simulink model "notch_filter"  (R2023a)
settings: configuration reference "config" (kept outside this file)
model workspace (MAT data in the model file):
  damp = Simulink.Parameter
  damp.Value = 10
  damp.DataType = 'double'
  damp.Complexity = 'real'
  damp.Dimensions = [1 1]
  dt = Simulink.Parameter
  dt.Value = 0.0001
  dt.DataType = 'double'
  dt.Complexity = 'real'
  dt.Dimensions = [1 1]
  freq = Simulink.Parameter
  freq.Value = 439
  freq.DataType = 'double'
  freq.Complexity = 'real'
  freq.Dimensions = [1 1]
  gmin = Simulink.Parameter
  gmin.Value = 100
  gmin.DataType = 'double'
  gmin.Complexity = 'real'
  gmin.Dimensions = [1 1]
settings Model: DataDictionary=model_config.sldd  ParameterArgumentNames=damp,dt,freq,gmin  Creator=GQR  LastModifiedBy=Administrator
settings ConfigSetRef: SourceName=config

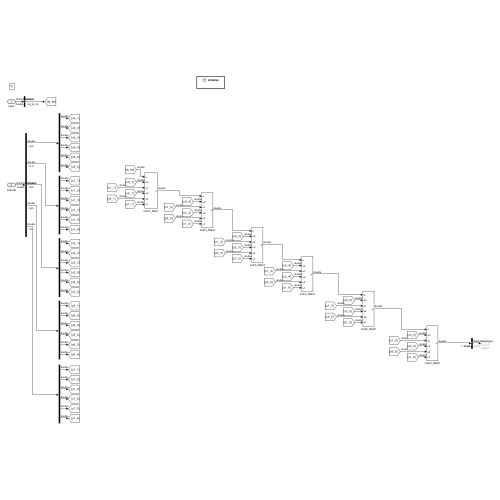
[thumbnail: Simulink's stored preview of the top-level diagram]
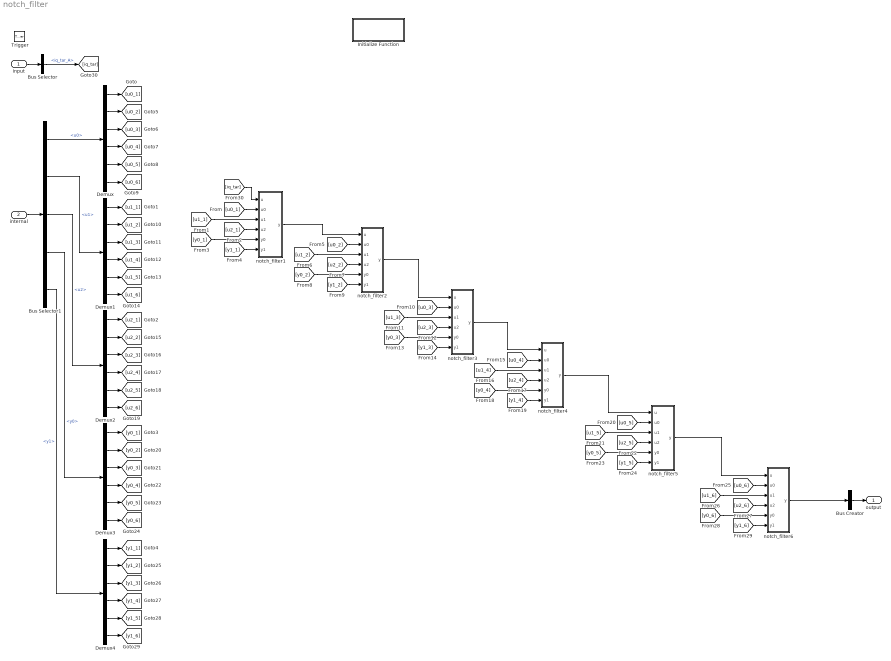
== system notch_filter ==
  input : Inport  OutDataTypeStr=Bus: NotchFilterInput  BusOutputAsStruct=on
  internal : Inport  Port=2  OutDataTypeStr=Bus: NotchFilterInternal  BusOutputAsStruct=on
  Trigger : TriggerPort  TriggerType=function-call  VariantControl=(inherit)  PortDimensions=1
  Bus Creator : BusCreator  Inputs=1  OutDataTypeStr=Bus: NotchFilterOutput  NonVirtualBus=on
      settings: InheritFromInputs=off
  Bus Selector : BusSelector  OutputSignals=iq_tar_A
  Bus Selector1 : BusSelector  OutputSignals=u0,u1,u2,y0,y1
  Demux{,1..4} (5 alike) : Demux  Outputs=6
  Initialize Function : Subsystem  TreatAsAtomicUnit=on
  notch_filter1 : Subsystem
  notch_filter2 : Subsystem
  notch_filter3 : Subsystem
  notch_filter4 : Subsystem
  notch_filter5 : Subsystem
  notch_filter6 : Subsystem
  output : Outport  OutDataTypeStr=Bus: NotchFilterOutput  BusOutputAsStruct=on
      settings: EnsureOutportIsVirtual=on
  wires:
  Demux4/6 -> [y1_6]
  Demux4/5 -> [y1_5]
  Demux1/1 -> [u1_1]
  internal/1 -> Bus Selector1/1
  Bus Selector1/5 -> Demux4/1  "<y1>"
  Demux2/2 -> [u2_2]
  input/1 -> Bus Selector/1
  Bus Selector1/4 -> Demux3/1  "<y0>"
  Bus Selector1/1 -> Demux/1  "<u0>"
  Bus Selector1/2 -> Demux1/1  "<u1>"
  Demux1/3 -> [u1_3]
  Bus Selector1/3 -> Demux2/1  "<u2>"
  Demux1/2 -> [u1_2]
  [u0_1] -> notch_filter1/2(u0)
  [u1_1] -> notch_filter1/3(u1)
  Bus Creator/1 -> output/1
  [u2_1] -> notch_filter1/4(u2)
  Demux3/6 -> [y0_6]
  Demux/2 -> [u0_2]
  [y1_1] -> notch_filter1/6(y1)
  [y0_1] -> notch_filter1/5(y0)
  Demux/1 -> [u0_1]
  Demux/3 -> [u0_3]
  Demux/4 -> [u0_4]
  Demux/5 -> [u0_5]
  Demux/6 -> [u0_6]
  Demux1/4 -> [u1_4]
  Demux1/5 -> [u1_5]
  Demux1/6 -> [u1_6]
  Demux2/6 -> [u2_6]
  Demux2/5 -> [u2_5]
  Demux2/1 -> [u2_1]
  Demux2/4 -> [u2_4]
  Demux2/3 -> [u2_3]
  Demux3/1 -> [y0_1]
  Demux3/3 -> [y0_3]
  Demux3/2 -> [y0_2]
  Demux3/5 -> [y0_5]
  Demux3/4 -> [y0_4]
  Demux4/2 -> [y1_2]
  Demux4/1 -> [y1_1]
  Demux4/4 -> [y1_4]
  Demux4/3 -> [y1_3]
  [y0_2] -> notch_filter2/5(y0)
  [y1_2] -> notch_filter2/6(y1)
  [u2_2] -> notch_filter2/4(u2)
  [u1_2] -> notch_filter2/3(u1)
  [u0_2] -> notch_filter2/2(u0)
  notch_filter1/1(y) -> notch_filter2/1(u)
  [u0_3] -> notch_filter3/2(u0)
  [u1_3] -> notch_filter3/3(u1)
  [u2_3] -> notch_filter3/4(u2)
  [y1_3] -> notch_filter3/6(y1)
  [y0_3] -> notch_filter3/5(y0)
  notch_filter2/1(y) -> notch_filter3/1(u)
  [y0_4] -> notch_filter4/5(y0)
  [y1_4] -> notch_filter4/6(y1)
  [u2_4] -> notch_filter4/4(u2)
  [u1_4] -> notch_filter4/3(u1)
  [u0_4] -> notch_filter4/2(u0)
  notch_filter3/1(y) -> notch_filter4/1(u)
  [u0_5] -> notch_filter5/2(u0)
  [u1_5] -> notch_filter5/3(u1)
  [u2_5] -> notch_filter5/4(u2)
  [y1_5] -> notch_filter5/6(y1)
  [y0_5] -> notch_filter5/5(y0)
  notch_filter4/1(y) -> notch_filter5/1(u)
  notch_filter5/1(y) -> notch_filter6/1(u)
  [y0_6] -> notch_filter6/5(y0)
  [y1_6] -> notch_filter6/6(y1)
  [u2_6] -> notch_filter6/4(u2)
  [u1_6] -> notch_filter6/3(u1)
  [u0_6] -> notch_filter6/2(u0)
  notch_filter6/1(y) -> Bus Creator/1
  Bus Selector/1 -> [iq_tar]  "<iq_tar_A>"
  [iq_tar] -> notch_filter1/1(u)

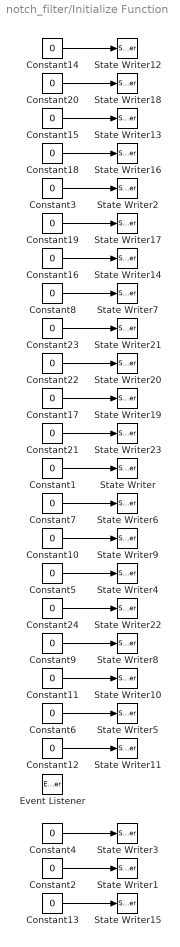
== system notch_filter/Initialize Function ==
  Constant{1..24} (24 alike) : Constant  Value=0  OutDataTypeStr=single
  Event Listener : EventListener  DisableCoverage=on  EventName=reset
  State Writer : StateWriter  StateOwnerBlock=../../notch_filter1/Delay  StateName=u_last
  State Writer1 : StateWriter  StateOwnerBlock=../../notch_filter1/Delay1  StateName=u_last
  State Writer10 : StateWriter  StateOwnerBlock=../../notch_filter3/Delay1  StateName=u_last
  State Writer11 : StateWriter  StateOwnerBlock=../../notch_filter3/Delay2  StateName=y_last
  State Writer12 : StateWriter  StateOwnerBlock=../../notch_filter4/Delay1  StateName=u_last
  State Writer13 : StateWriter  StateOwnerBlock=../../notch_filter4/Delay2  StateName=y_last
  State Writer14 : StateWriter  StateOwnerBlock=../../notch_filter4/Delay  StateName=u_last
  State Writer15 : StateWriter  StateOwnerBlock=../../notch_filter4/Delay3  StateName=y_last
  State Writer16 : StateWriter  StateOwnerBlock=../../notch_filter5/Delay1  StateName=u_last
  State Writer17 : StateWriter  StateOwnerBlock=../../notch_filter5/Delay2  StateName=y_last
  State Writer18 : StateWriter  StateOwnerBlock=../../notch_filter5/Delay  StateName=u_last
  State Writer19 : StateWriter  StateOwnerBlock=../../notch_filter5/Delay3  StateName=y_last
  State Writer2 : StateWriter  StateOwnerBlock=../../notch_filter1/Delay2  StateName=y_last
  State Writer20 : StateWriter  StateOwnerBlock=../../notch_filter6/Delay1  StateName=u_last
  State Writer21 : StateWriter  StateOwnerBlock=../../notch_filter6/Delay2  StateName=y_last
  State Writer22 : StateWriter  StateOwnerBlock=../../notch_filter6/Delay  StateName=u_last
  State Writer23 : StateWriter  StateOwnerBlock=../../notch_filter6/Delay3  StateName=y_last
  State Writer3 : StateWriter  StateOwnerBlock=../../notch_filter1/Delay3  StateName=y_last
  State Writer4 : StateWriter  StateOwnerBlock=../../notch_filter2/Delay  StateName=u_last
  State Writer5 : StateWriter  StateOwnerBlock=../../notch_filter2/Delay3  StateName=y_last
  State Writer6 : StateWriter  StateOwnerBlock=../../notch_filter2/Delay1  StateName=u_last
  State Writer7 : StateWriter  StateOwnerBlock=../../notch_filter2/Delay2  StateName=y_last
  State Writer8 : StateWriter  StateOwnerBlock=../../notch_filter3/Delay  StateName=u_last
  State Writer9 : StateWriter  StateOwnerBlock=../../notch_filter3/Delay3  StateName=y_last
  wires:
  Constant15/1 -> State Writer13/1
  Constant12/1 -> State Writer11/1
  Constant14/1 -> State Writer12/1
  Constant20/1 -> State Writer18/1
  Constant18/1 -> State Writer16/1
  Constant3/1 -> State Writer2/1
  Constant8/1 -> State Writer7/1
  Constant19/1 -> State Writer17/1
  Constant16/1 -> State Writer14/1
  Constant23/1 -> State Writer21/1
  Constant22/1 -> State Writer20/1
  Constant17/1 -> State Writer19/1
  Constant21/1 -> State Writer23/1
  Constant1/1 -> State Writer/1
  Constant7/1 -> State Writer6/1
  Constant10/1 -> State Writer9/1
  Constant2/1 -> State Writer1/1
  Constant5/1 -> State Writer4/1
  Constant24/1 -> State Writer22/1
  Constant9/1 -> State Writer8/1
  Constant11/1 -> State Writer10/1
  Constant6/1 -> State Writer5/1
  Constant4/1 -> State Writer3/1
  Constant13/1 -> State Writer15/1

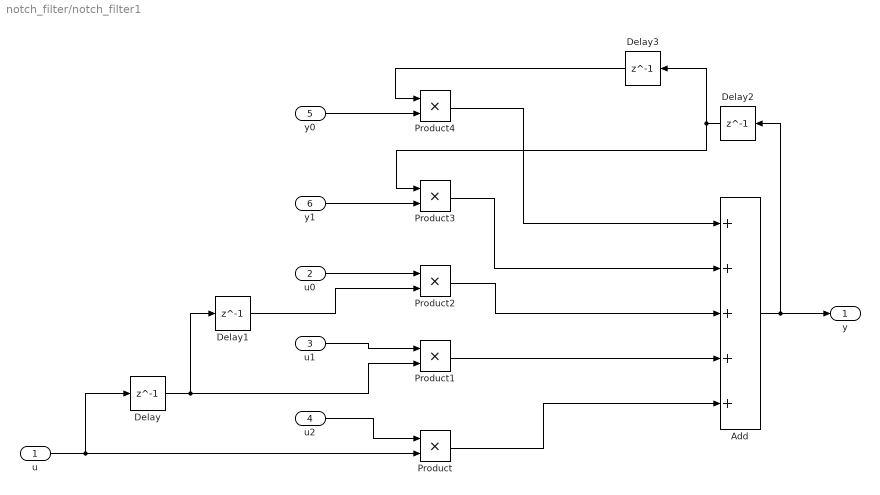
== system notch_filter/notch_filter1 ==
  u : Inport
  u0 : Inport  Port=2
  u1 : Inport  Port=3
  u2 : Inport  Port=4
  y0 : Inport  Port=5
  y1 : Inport  Port=6
  Add : Sum  Inputs=+++++
  Delay : Delay  DelayLength=1  StateName=u_last
  Delay1 : Delay  DelayLength=1  StateName=u_last
  Delay2 : Delay  DelayLength=1  StateName=y_last
  Delay3 : Delay  DelayLength=1  StateName=y_last
  Product{,1..4} (5 alike) : Product
  y : Outport
  wires:
  u2/1 -> Product/1
  Product3/1 -> Add/2
  y1/1 -> Product3/2
  Delay3/1 -> Product4/1
  u/1 -> Delay/1, Product/2
  Delay2/1 -> Product3/1, Delay3/1
  Product4/1 -> Add/1
  u0/1 -> Product2/1
  Product1/1 -> Add/4
  Product2/1 -> Add/3
  y0/1 -> Product4/2
  Delay/1 -> Product1/2, Delay1/1
  Add/1 -> y/1, Delay2/1
  Delay1/1 -> Product2/2
  u1/1 -> Product1/1
  Product/1 -> Add/5

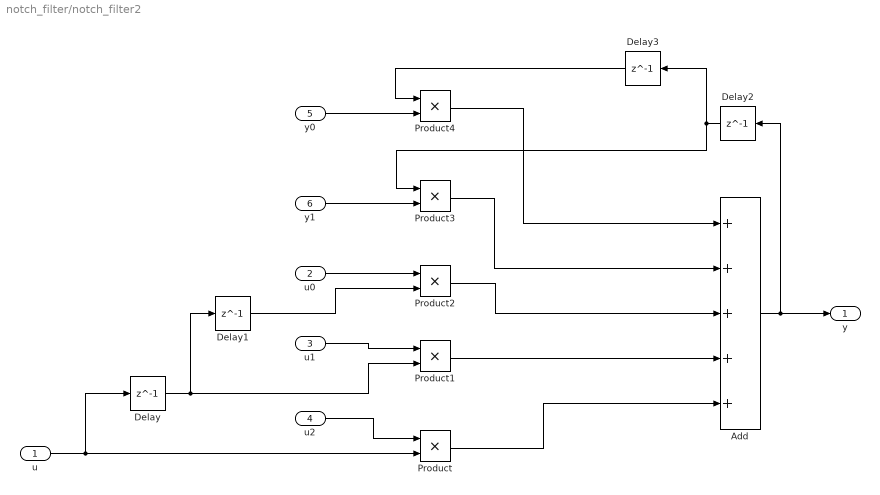
== system notch_filter/notch_filter2 ==
  u : Inport
  u0 : Inport  Port=2
  u1 : Inport  Port=3
  u2 : Inport  Port=4
  y0 : Inport  Port=5
  y1 : Inport  Port=6
  Add : Sum  Inputs=+++++
  Delay : Delay  DelayLength=1  StateName=u_last
  Delay1 : Delay  DelayLength=1  StateName=u_last
  Delay2 : Delay  DelayLength=1  StateName=y_last
  Delay3 : Delay  DelayLength=1  StateName=y_last
  Product{,1..4} (5 alike) : Product
  y : Outport
  wires:
  Product/1 -> Add/5
  u1/1 -> Product1/1
  Delay1/1 -> Product2/2
  Add/1 -> Delay2/1, y/1
  Delay/1 -> Delay1/1, Product1/2
  y0/1 -> Product4/2
  Product2/1 -> Add/3
  Product1/1 -> Add/4
  u0/1 -> Product2/1
  Product4/1 -> Add/1
  Delay2/1 -> Delay3/1, Product3/1
  u/1 -> Product/2, Delay/1
  Delay3/1 -> Product4/1
  y1/1 -> Product3/2
  Product3/1 -> Add/2
  u2/1 -> Product/1

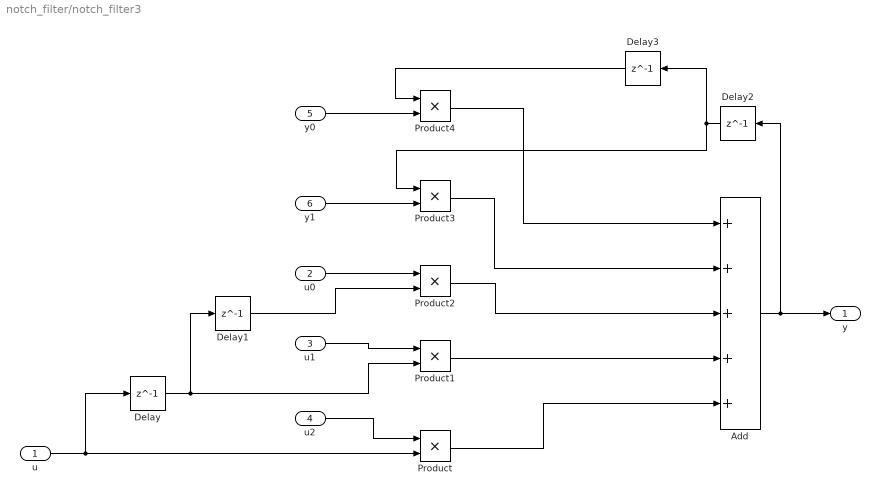
== system notch_filter/notch_filter3 ==
  u : Inport
  u0 : Inport  Port=2
  u1 : Inport  Port=3
  u2 : Inport  Port=4
  y0 : Inport  Port=5
  y1 : Inport  Port=6
  Add : Sum  Inputs=+++++
  Delay : Delay  DelayLength=1  StateName=u_last
  Delay1 : Delay  DelayLength=1  StateName=u_last
  Delay2 : Delay  DelayLength=1  StateName=y_last
  Delay3 : Delay  DelayLength=1  StateName=y_last
  Product{,1..4} (5 alike) : Product
  y : Outport
  wires:
  u2/1 -> Product/1
  Product3/1 -> Add/2
  y1/1 -> Product3/2
  Delay3/1 -> Product4/1
  u/1 -> Delay/1, Product/2
  Delay2/1 -> Product3/1, Delay3/1
  Product4/1 -> Add/1
  u0/1 -> Product2/1
  Product1/1 -> Add/4
  Product2/1 -> Add/3
  y0/1 -> Product4/2
  Delay/1 -> Product1/2, Delay1/1
  Add/1 -> y/1, Delay2/1
  Delay1/1 -> Product2/2
  u1/1 -> Product1/1
  Product/1 -> Add/5

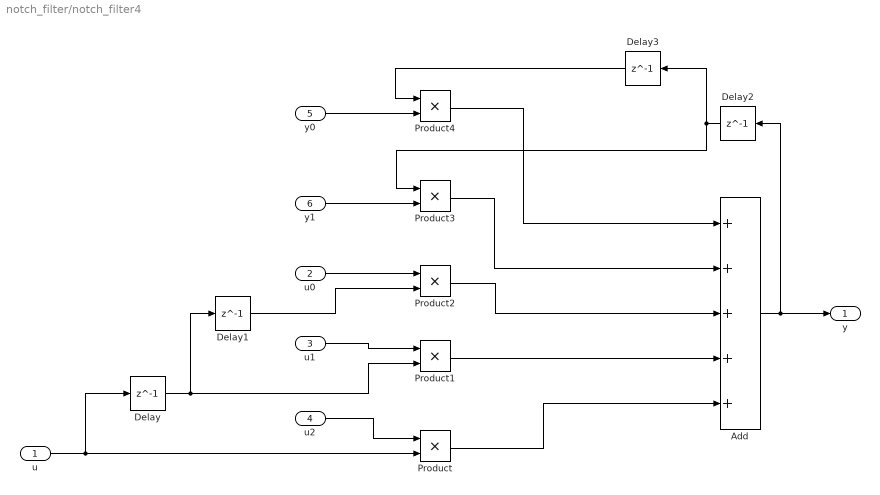
== system notch_filter/notch_filter4 ==
  u : Inport
  u0 : Inport  Port=2
  u1 : Inport  Port=3
  u2 : Inport  Port=4
  y0 : Inport  Port=5
  y1 : Inport  Port=6
  Add : Sum  Inputs=+++++
  Delay : Delay  DelayLength=1  StateName=u_last
  Delay1 : Delay  DelayLength=1  StateName=u_last
  Delay2 : Delay  DelayLength=1  StateName=y_last
  Delay3 : Delay  DelayLength=1  StateName=y_last
  Product{,1..4} (5 alike) : Product
  y : Outport
  wires:
  Product/1 -> Add/5
  u1/1 -> Product1/1
  Delay1/1 -> Product2/2
  Add/1 -> Delay2/1, y/1
  Delay/1 -> Delay1/1, Product1/2
  y0/1 -> Product4/2
  Product2/1 -> Add/3
  Product1/1 -> Add/4
  u0/1 -> Product2/1
  Product4/1 -> Add/1
  Delay2/1 -> Delay3/1, Product3/1
  u/1 -> Product/2, Delay/1
  Delay3/1 -> Product4/1
  y1/1 -> Product3/2
  Product3/1 -> Add/2
  u2/1 -> Product/1

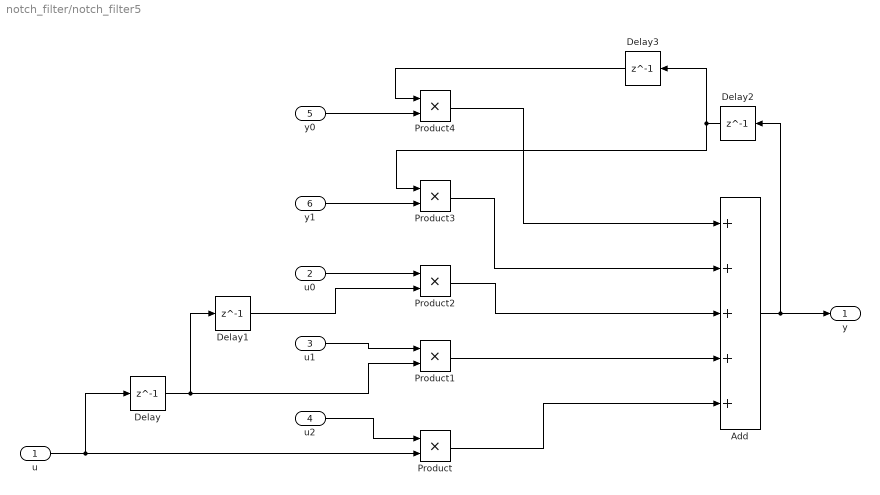
== system notch_filter/notch_filter5 ==
  u : Inport
  u0 : Inport  Port=2
  u1 : Inport  Port=3
  u2 : Inport  Port=4
  y0 : Inport  Port=5
  y1 : Inport  Port=6
  Add : Sum  Inputs=+++++
  Delay : Delay  DelayLength=1  StateName=u_last
  Delay1 : Delay  DelayLength=1  StateName=u_last
  Delay2 : Delay  DelayLength=1  StateName=y_last
  Delay3 : Delay  DelayLength=1  StateName=y_last
  Product{,1..4} (5 alike) : Product
  y : Outport
  wires:
  u2/1 -> Product/1
  Product3/1 -> Add/2
  y1/1 -> Product3/2
  Delay3/1 -> Product4/1
  u/1 -> Delay/1, Product/2
  Delay2/1 -> Product3/1, Delay3/1
  Product4/1 -> Add/1
  u0/1 -> Product2/1
  Product1/1 -> Add/4
  Product2/1 -> Add/3
  y0/1 -> Product4/2
  Delay/1 -> Product1/2, Delay1/1
  Add/1 -> y/1, Delay2/1
  Delay1/1 -> Product2/2
  u1/1 -> Product1/1
  Product/1 -> Add/5

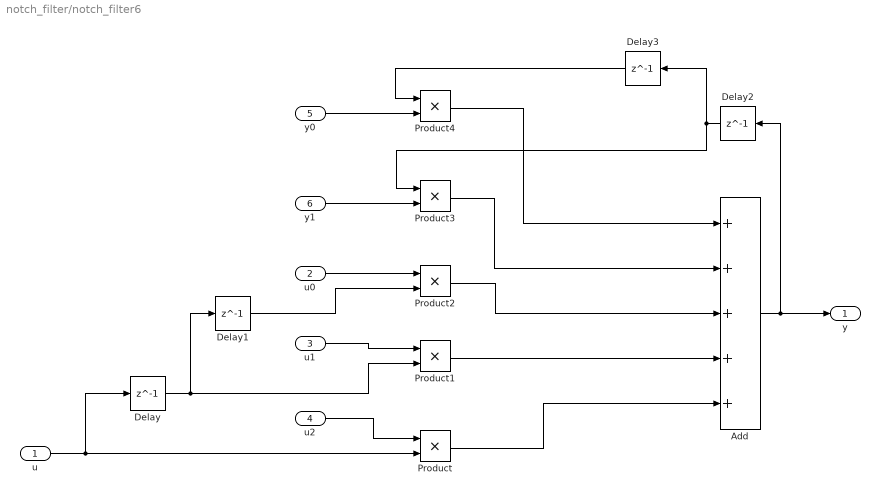
== system notch_filter/notch_filter6 ==
  u : Inport
  u0 : Inport  Port=2
  u1 : Inport  Port=3
  u2 : Inport  Port=4
  y0 : Inport  Port=5
  y1 : Inport  Port=6
  Add : Sum  Inputs=+++++
  Delay : Delay  DelayLength=1  StateName=u_last
  Delay1 : Delay  DelayLength=1  StateName=u_last
  Delay2 : Delay  DelayLength=1  StateName=y_last
  Delay3 : Delay  DelayLength=1  StateName=y_last
  Product{,1..4} (5 alike) : Product
  y : Outport
  wires:
  Product/1 -> Add/5
  u1/1 -> Product1/1
  Delay1/1 -> Product2/2
  Add/1 -> Delay2/1, y/1
  Delay/1 -> Delay1/1, Product1/2
  y0/1 -> Product4/2
  Product2/1 -> Add/3
  Product1/1 -> Add/4
  u0/1 -> Product2/1
  Product4/1 -> Add/1
  Delay2/1 -> Delay3/1, Product3/1
  u/1 -> Product/2, Delay/1
  Delay3/1 -> Product4/1
  y1/1 -> Product3/2
  Product3/1 -> Add/2
  u2/1 -> Product/1
